simulink model "HANcoder_E407_GTSync_v4"  (R2018b)
settings: Solver=FixedStepDiscrete  StartTime=0.0  StopTime=1  FixedStep=0.01  RelTol=1e-3
PreLoadFcn:
  | librarySetup
  | eval([bdroot,'_startup']) %Calling [modelName]_startup.m
values from neighbouring files (symbols this model uses):
  basic_cycle_duration = TM12 + COMP_duration    (= 495)    [HANcoder_E407_GTSync_v4_startup.m]
  COM_Period = 100    [HANcoder_E407_GTSync_v4_startup.m]
  COM_Phase = COM_Period/2    (= 50)    [HANcoder_E407_GTSync_v4_startup.m]
  comm_delay_estimation = 20    [HANcoder_E407_GTSync_v4_startup.m]
  frequency_IRQ = 20    [HANcoder_E407_GTSync_v4_startup.m]
  HANtuneOverride = Simulink.Parameter    [HANcoder_E407_GTSync_v4_startup.m]
  idle_time_init = basic_cycle_duration*matrix_rows    (= 990)    [HANcoder_E407_GTSync_v4_startup.m]
  LED_ticks_toggle = 10000    [HANcoder_E407_GTSync_v4_startup.m]
  Master_Role = 1    [HANcoder_E407_GTSync_v4_startup.m]
  matrix_rows = 2    [HANcoder_E407_GTSync_v4_startup.m]
  Slave_Role = 2    [HANcoder_E407_GTSync_v4_startup.m]
  Sync_ID = 1    [HANcoder_E407_GTSync_v4_startup.m]
  time_difference_threshold = 500    [HANcoder_E407_GTSync_v4_startup.m]
  TM0 = basic_cycle_start    (= 5)    [HANcoder_E407_GTSync_v4_startup.m]
  TM1 = TM0 + COMM_duration    (= 105)    [HANcoder_E407_GTSync_v4_startup.m]
  TM10 = TM9  + COMP_duration    (= 465)    [HANcoder_E407_GTSync_v4_startup.m]
  TM11 = TM10 + COMP_duration    (= 475)    [HANcoder_E407_GTSync_v4_startup.m]
  TM12 = TM11 + COMP_duration    (= 485)    [HANcoder_E407_GTSync_v4_startup.m]
  TM2 = TM1 + COMP_duration    (= 115)    [HANcoder_E407_GTSync_v4_startup.m]
  TM3 = TM2 + COMP_duration    (= 125)    [HANcoder_E407_GTSync_v4_startup.m]
  TM4 = TM3 + COMM_duration    (= 225)    [HANcoder_E407_GTSync_v4_startup.m]
  TM5 = TM4 + COMP_duration    (= 235)    [HANcoder_E407_GTSync_v4_startup.m]
  TM6 = TM5 + COMM_duration    (= 335)    [HANcoder_E407_GTSync_v4_startup.m]
  TM7 = TM6 + COMP_duration    (= 345)    [HANcoder_E407_GTSync_v4_startup.m]
  TM8 = TM7 + COMM_duration    (= 445)    [HANcoder_E407_GTSync_v4_startup.m]
  TM9 = TM8  + COMP_duration    (= 455)    [HANcoder_E407_GTSync_v4_startup.m]
  Vote1_ID = 12    [HANcoder_E407_GTSync_v4_startup.m]
  Vote2_ID = 22    [HANcoder_E407_GTSync_v4_startup.m]
  Vote3_ID = 32    [HANcoder_E407_GTSync_v4_startup.m]
  wrap_up_threshold = basic_cycle_duration - time_difference_threshold*10    (= -4505)    [HANcoder_E407_GTSync_v4_startup.m]
undefined symbols (not defined in the file or in its folder): A0, A1, CON2
libraries: HANcoder_STM32_Target x22, simulink x3, hdlsllib x2, simulink_extras x1
(part 3 of 5)

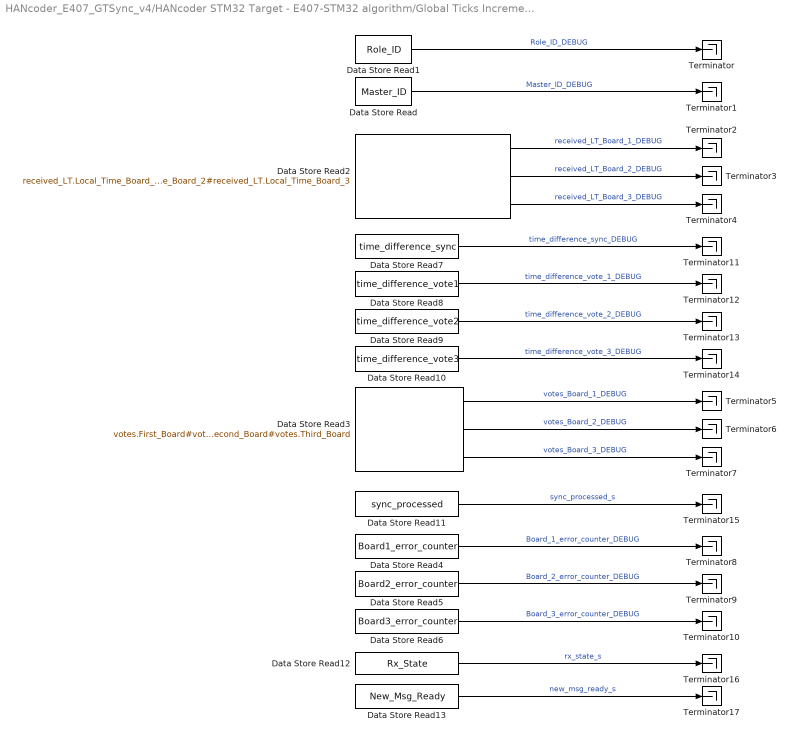
== system HANcoder_E407_GTSync_v4/HANcoder STM32 Target - E407-STM32 algorithm/Global Ticks Increment/CAN Management/Matrix Cycle Manager/Matrix_Cycle_Observation_DEBUG ==
  Data Store Read : DataStoreRead  DataStoreName=Master_ID
  Data Store Read1 : DataStoreRead  DataStoreName=Role_ID
  Data Store Read10 : DataStoreRead  DataStoreName=time_difference_vote3
  Data Store Read11 : DataStoreRead  DataStoreName=sync_processed
  Data Store Read12 : DataStoreRead  DataStoreName=Rx_State
  Data Store Read13 : DataStoreRead  DataStoreName=New_Msg_Ready
  Data Store Read2 : DataStoreRead  DataStoreName=received_LT  DataStoreElements=received_LT.Local_Time_Board_1#received_LT.Local_Time_Board_2#received_LT.Local_Time_Board_3
  Data Store Read3 : DataStoreRead  DataStoreName=votes  DataStoreElements=votes.First_Board#votes.Second_Board#votes.Third_Board
  Data Store Read4 : DataStoreRead  DataStoreName=Board1_error_counter
  Data Store Read5 : DataStoreRead  DataStoreName=Board2_error_counter
  Data Store Read6 : DataStoreRead  DataStoreName=Board3_error_counter
  Data Store Read7 : DataStoreRead  DataStoreName=time_difference_sync
  Data Store Read8 : DataStoreRead  DataStoreName=time_difference_vote1
  Data Store Read9 : DataStoreRead  DataStoreName=time_difference_vote2
  Terminator{,1..17} (18 alike) : Terminator
  wires:
  Data Store Read1/1 -> Terminator/1  "Role_ID_DEBUG"
  Data Store Read/1 -> Terminator1/1  "Master_ID_DEBUG"
  Data Store Read2/1 -> Terminator2/1  "received_LT_Board_1_DEBUG"
  Data Store Read2/2 -> Terminator3/1  "received_LT_Board_2_DEBUG"
  Data Store Read2/3 -> Terminator4/1  "received_LT_Board_3_DEBUG"
  Data Store Read3/1 -> Terminator5/1  "votes_Board_1_DEBUG"
  Data Store Read3/2 -> Terminator6/1  "votes_Board_2_DEBUG"
  Data Store Read3/3 -> Terminator7/1  "votes_Board_3_DEBUG"
  Data Store Read4/1 -> Terminator8/1  "Board_1_error_counter_DEBUG"
  Data Store Read5/1 -> Terminator9/1  "Board_2_error_counter_DEBUG"
  Data Store Read6/1 -> Terminator10/1  "Board_3_error_counter_DEBUG"
  Data Store Read7/1 -> Terminator11/1  "time_difference_sync_DEBUG"
  Data Store Read8/1 -> Terminator12/1  "time_difference_vote_1_DEBUG"
  Data Store Read9/1 -> Terminator13/1  "time_difference_vote_2_DEBUG"
  Data Store Read10/1 -> Terminator14/1  "time_difference_vote_3_DEBUG"
  Data Store Read11/1 -> Terminator15/1  "sync_processed_s"
  Data Store Read12/1 -> Terminator16/1  "rx_state_s"
  Data Store Read13/1 -> Terminator17/1  "new_msg_ready_s"

== system HANcoder_E407_GTSync_v4/HANcoder STM32 Target - E407-STM32 algorithm/Global Ticks Increment/CAN Recieve/RxID_CAN/Sync_ID_CAN ==
  Enable : EnablePort
  CAN receive : Subsystem  Tag=HANcoder_TARGET_STM32_E407  AncestorBlock=HANcoder_STM32_Target/STM32-E407/CAN/CAN/CAN receive  mask(CAN receive){canBus=CAN 2, outputNumber=8, dataType=uint8, byteOrder=off, tsamp=-1}
      mask prompts: canBus "CAN channel"; outputNumber "Output ports"; dataType "Output datatype"; byteOrder "Byte order: Checked = MSB first, unchecked = LSB first."; tsamp "Sample time"
      mask help:
      | Function
      | ==========
      | Receive the newest message from the specified CAN channel.
      |
      | Parameters
      | ==========
      | CAN channel:             The CAN channel to send the message on.
      | Output ports:             The amount of output ports
      | Output datatype:       The datatype of the output ports
      | Byte order:                 Select MSB or LSB first
      | Sample time:              -1 or divisible by base sample time [seconds]
      |
      | Input
      | ==========
      | Port 1:                       CAN ID(uint32) in hexadecimal ie: hex2dec('0a')
      |
      | Output
      | ==========
      | Port 1:                       Checks for new message(int8)
      | Port 2..9                     Message data
      mask init:
      | sfcn_can_receive_mcb(canBus, outputNumber, dataType, byteOrder)
      settings: MoveFcn=drawLogos
      mask Help: web('sfcn_can_receive.html');
      mask TypeOptions canBus: CAN 1 | CAN 2
      mask TypeOptions dataType: int8 | uint8 | int16 | uint16 | int32 | uint32 | boolean
      mask Display:
      | fprintf('Receive on\nCAN %x', canBus);
      | port_label('output', 1, 'new');
      | port_label('input', 1, 'ID');patch([135 141 141],[8 14 2],[1 0 0]);patch([143 143 149],[14 2 8],[0 0 0.35]);
  Constant : Constant  Value=Sync_ID  OutDataTypeStr=uint32
  CAN_new : Outport  OutputWhenDisabled=reset  InitialOutput=0
  Out2 : Outport  Port=2  OutputWhenDisabled=reset  InitialOutput=0
  Out3 : Outport  Port=3  OutputWhenDisabled=reset  InitialOutput=0
  Out4 : Outport  Port=4  OutputWhenDisabled=reset  InitialOutput=0
  Out5 : Outport  Port=5  OutputWhenDisabled=reset  InitialOutput=0
  Out6 : Outport  Port=6  OutputWhenDisabled=reset  InitialOutput=0
  Out7 : Outport  Port=7  OutputWhenDisabled=reset  InitialOutput=0
  Out8 : Outport  Port=8  OutputWhenDisabled=reset  InitialOutput=0
  Out9 : Outport  Port=9  OutputWhenDisabled=reset  InitialOutput=0
  wires:
  CAN receive/1(Out1) -> CAN_new/1
  CAN receive/8(Out8) -> Out8/1
  CAN receive/3(Out3) -> Out3/1
  Constant/1 -> CAN receive/1(In1)
  CAN receive/2(Out2) -> Out2/1
  CAN receive/6(Out6) -> Out6/1
  CAN receive/7(Out7) -> Out7/1
  CAN receive/4(Out4) -> Out4/1
  CAN receive/5(Out5) -> Out5/1
  CAN receive/9(Out9) -> Out9/1

== system HANcoder_E407_GTSync_v4/HANcoder STM32 Target - E407-STM32 algorithm/Global Ticks Increment/CAN Recieve/RxID_CAN/Vote1_ID_CAN ==
  Enable : EnablePort
  CAN receive : Subsystem  Tag=HANcoder_TARGET_STM32_E407  AncestorBlock=HANcoder_STM32_Target/STM32-E407/CAN/CAN/CAN receive  mask(CAN receive){canBus=CAN 2, outputNumber=8, dataType=uint8, byteOrder=off, tsamp=-1}
      mask prompts: canBus "CAN channel"; outputNumber "Output ports"; dataType "Output datatype"; byteOrder "Byte order: Checked = MSB first, unchecked = LSB first."; tsamp "Sample time"
      mask help:
      | Function
      | ==========
      | Receive the newest message from the specified CAN channel.
      |
      | Parameters
      | ==========
      | CAN channel:             The CAN channel to send the message on.
      | Output ports:             The amount of output ports
      | Output datatype:       The datatype of the output ports
      | Byte order:                 Select MSB or LSB first
      | Sample time:              -1 or divisible by base sample time [seconds]
      |
      | Input
      | ==========
      | Port 1:                       CAN ID(uint32) in hexadecimal ie: hex2dec('0a')
      |
      | Output
      | ==========
      | Port 1:                       Checks for new message(int8)
      | Port 2..9                     Message data
      mask init:
      | sfcn_can_receive_mcb(canBus, outputNumber, dataType, byteOrder)
      settings: MoveFcn=drawLogos
      mask Help: web('sfcn_can_receive.html');
      mask TypeOptions canBus: CAN 1 | CAN 2
      mask TypeOptions dataType: int8 | uint8 | int16 | uint16 | int32 | uint32 | boolean
      mask Display:
      | fprintf('Receive on\nCAN %x', canBus);
      | port_label('output', 1, 'new');
      | port_label('input', 1, 'ID');patch([135 141 141],[8 14 2],[1 0 0]);patch([143 143 149],[14 2 8],[0 0 0.35]);
  Constant : Constant  Value=Vote1_ID  OutDataTypeStr=uint32
  CAN_new : Outport  OutputWhenDisabled=reset  InitialOutput=0
  Out2 : Outport  Port=2  OutputWhenDisabled=reset  InitialOutput=0
  Out3 : Outport  Port=3  OutputWhenDisabled=reset  InitialOutput=0
  Out4 : Outport  Port=4  OutputWhenDisabled=reset  InitialOutput=0
  Out5 : Outport  Port=5  OutputWhenDisabled=reset  InitialOutput=0
  Out6 : Outport  Port=6  OutputWhenDisabled=reset  InitialOutput=0
  Out7 : Outport  Port=7  OutputWhenDisabled=reset  InitialOutput=0
  Out8 : Outport  Port=8  OutputWhenDisabled=reset  InitialOutput=0
  Out9 : Outport  Port=9  OutputWhenDisabled=reset  InitialOutput=0
  wires:
  CAN receive/9(Out9) -> Out9/1
  CAN receive/5(Out5) -> Out5/1
  CAN receive/4(Out4) -> Out4/1
  CAN receive/7(Out7) -> Out7/1
  CAN receive/6(Out6) -> Out6/1
  CAN receive/2(Out2) -> Out2/1
  Constant/1 -> CAN receive/1(In1)
  CAN receive/3(Out3) -> Out3/1
  CAN receive/8(Out8) -> Out8/1
  CAN receive/1(Out1) -> CAN_new/1

== system HANcoder_E407_GTSync_v4/HANcoder STM32 Target - E407-STM32 algorithm/Global Ticks Increment/CAN Recieve/RxID_CAN/Vote2_ID_CAN ==
  Enable : EnablePort
  CAN receive : Subsystem  Tag=HANcoder_TARGET_STM32_E407  AncestorBlock=HANcoder_STM32_Target/STM32-E407/CAN/CAN/CAN receive  mask(CAN receive){canBus=CAN 2, outputNumber=8, dataType=uint8, byteOrder=off, tsamp=-1}
      mask prompts: canBus "CAN channel"; outputNumber "Output ports"; dataType "Output datatype"; byteOrder "Byte order: Checked = MSB first, unchecked = LSB first."; tsamp "Sample time"
      mask help:
      | Function
      | ==========
      | Receive the newest message from the specified CAN channel.
      |
      | Parameters
      | ==========
      | CAN channel:             The CAN channel to send the message on.
      | Output ports:             The amount of output ports
      | Output datatype:       The datatype of the output ports
      | Byte order:                 Select MSB or LSB first
      | Sample time:              -1 or divisible by base sample time [seconds]
      |
      | Input
      | ==========
      | Port 1:                       CAN ID(uint32) in hexadecimal ie: hex2dec('0a')
      |
      | Output
      | ==========
      | Port 1:                       Checks for new message(int8)
      | Port 2..9                     Message data
      mask init:
      | sfcn_can_receive_mcb(canBus, outputNumber, dataType, byteOrder)
      settings: MoveFcn=drawLogos
      mask Help: web('sfcn_can_receive.html');
      mask TypeOptions canBus: CAN 1 | CAN 2
      mask TypeOptions dataType: int8 | uint8 | int16 | uint16 | int32 | uint32 | boolean
      mask Display:
      | fprintf('Receive on\nCAN %x', canBus);
      | port_label('output', 1, 'new');
      | port_label('input', 1, 'ID');patch([135 141 141],[8 14 2],[1 0 0]);patch([143 143 149],[14 2 8],[0 0 0.35]);
  Constant : Constant  Value=Vote2_ID  OutDataTypeStr=uint32
  CAN_new : Outport  OutputWhenDisabled=reset  InitialOutput=0
  Out2 : Outport  Port=2  OutputWhenDisabled=reset  InitialOutput=0
  Out3 : Outport  Port=3  OutputWhenDisabled=reset  InitialOutput=0
  Out4 : Outport  Port=4  OutputWhenDisabled=reset  InitialOutput=0
  Out5 : Outport  Port=5  OutputWhenDisabled=reset  InitialOutput=0
  Out6 : Outport  Port=6  OutputWhenDisabled=reset  InitialOutput=0
  Out7 : Outport  Port=7  OutputWhenDisabled=reset  InitialOutput=0
  Out8 : Outport  Port=8  OutputWhenDisabled=reset  InitialOutput=0
  Out9 : Outport  Port=9  OutputWhenDisabled=reset  InitialOutput=0
  wires:
  CAN receive/1(Out1) -> CAN_new/1
  CAN receive/8(Out8) -> Out8/1
  CAN receive/3(Out3) -> Out3/1
  Constant/1 -> CAN receive/1(In1)
  CAN receive/2(Out2) -> Out2/1
  CAN receive/6(Out6) -> Out6/1
  CAN receive/7(Out7) -> Out7/1
  CAN receive/4(Out4) -> Out4/1
  CAN receive/5(Out5) -> Out5/1
  CAN receive/9(Out9) -> Out9/1

== system HANcoder_E407_GTSync_v4/HANcoder STM32 Target - E407-STM32 algorithm/Global Ticks Increment/CAN Recieve/RxID_CAN/Vote3_ID_CAN ==
  Enable : EnablePort
  CAN receive : Subsystem  Tag=HANcoder_TARGET_STM32_E407  AncestorBlock=HANcoder_STM32_Target/STM32-E407/CAN/CAN/CAN receive  mask(CAN receive){canBus=CAN 2, outputNumber=8, dataType=uint8, byteOrder=off, tsamp=-1}
      mask prompts: canBus "CAN channel"; outputNumber "Output ports"; dataType "Output datatype"; byteOrder "Byte order: Checked = MSB first, unchecked = LSB first."; tsamp "Sample time"
      mask help:
      | Function
      | ==========
      | Receive the newest message from the specified CAN channel.
      |
      | Parameters
      | ==========
      | CAN channel:             The CAN channel to send the message on.
      | Output ports:             The amount of output ports
      | Output datatype:       The datatype of the output ports
      | Byte order:                 Select MSB or LSB first
      | Sample time:              -1 or divisible by base sample time [seconds]
      |
      | Input
      | ==========
      | Port 1:                       CAN ID(uint32) in hexadecimal ie: hex2dec('0a')
      |
      | Output
      | ==========
      | Port 1:                       Checks for new message(int8)
      | Port 2..9                     Message data
      mask init:
      | sfcn_can_receive_mcb(canBus, outputNumber, dataType, byteOrder)
      settings: MoveFcn=drawLogos
      mask Help: web('sfcn_can_receive.html');
      mask TypeOptions canBus: CAN 1 | CAN 2
      mask TypeOptions dataType: int8 | uint8 | int16 | uint16 | int32 | uint32 | boolean
      mask Display:
      | fprintf('Receive on\nCAN %x', canBus);
      | port_label('output', 1, 'new');
      | port_label('input', 1, 'ID');patch([135 141 141],[8 14 2],[1 0 0]);patch([143 143 149],[14 2 8],[0 0 0.35]);
  Constant : Constant  Value=Vote3_ID  OutDataTypeStr=uint32
  CAN_new : Outport  OutputWhenDisabled=reset  InitialOutput=0
  Out2 : Outport  Port=2  OutputWhenDisabled=reset  InitialOutput=0
  Out3 : Outport  Port=3  OutputWhenDisabled=reset  InitialOutput=0
  Out4 : Outport  Port=4  OutputWhenDisabled=reset  InitialOutput=0
  Out5 : Outport  Port=5  OutputWhenDisabled=reset  InitialOutput=0
  Out6 : Outport  Port=6  OutputWhenDisabled=reset  InitialOutput=0
  Out7 : Outport  Port=7  OutputWhenDisabled=reset  InitialOutput=0
  Out8 : Outport  Port=8  OutputWhenDisabled=reset  InitialOutput=0
  Out9 : Outport  Port=9  OutputWhenDisabled=reset  InitialOutput=0
  wires:
  CAN receive/9(Out9) -> Out9/1
  CAN receive/5(Out5) -> Out5/1
  CAN receive/4(Out4) -> Out4/1
  CAN receive/7(Out7) -> Out7/1
  CAN receive/6(Out6) -> Out6/1
  CAN receive/2(Out2) -> Out2/1
  Constant/1 -> CAN receive/1(In1)
  CAN receive/3(Out3) -> Out3/1
  CAN receive/8(Out8) -> Out8/1
  CAN receive/1(Out1) -> CAN_new/1

== system HANcoder_E407_GTSync_v4/HANcoder STM32 Target - E407-STM32 algorithm/Global Ticks Increment/CAN Recieve/Update message buffers/UINT8 to UINT16 ==
  In1 : Inport
  In2 : Inport  Port=2
  Bit Shift : hdlsllib/Logic and Bit Operations/Bit Shift  mode=Shift Left Logical  N=8
      settings: SourceProductName=HDL Coder  SourceProductBaseCode=HD
  Cast1 : DataTypeConversion  OutDataTypeStr=uint16
  Cast4 : DataTypeConversion  OutDataTypeStr=uint16
  Sum1 : Sum
  Out1 : Outport
  wires:
  In1/1 -> Cast4/1
  Bit Shift/1 -> Sum1/2
  Cast1/1 -> Bit Shift/1
  In2/1 -> Cast1/1
  Sum1/1 -> Out1/1
  Cast4/1 -> Sum1/1

== system HANcoder_E407_GTSync_v4/HANcoder STM32 Target - E407-STM32 algorithm/Global Ticks Increment/CAN Management/Initialization/Delay/Initializaton_Observation_DEBUG ==
  Data Store Read : DataStoreRead  DataStoreName=Initialization_flag
  Data Store Read1 : DataStoreRead  DataStoreName=Delay_Counter
  Data Store Read2 : DataStoreRead  DataStoreName=New_Msg_Ready
  Data Store Read3 : DataStoreRead  DataStoreName=Initialization_Timeout
  Data Store Read5 : DataStoreRead  DataStoreName=basic_cycle_count
  Terminator{,1..3,5} (5 alike) : Terminator
  wires:
  Data Store Read3/1 -> Terminator3/1  "initialization_timeout_DEBUG"
  Data Store Read1/1 -> Terminator1/1  "delay_counter_DEBUG"
  Data Store Read/1 -> Terminator/1  "initialization_flag_DEBUG"
  Data Store Read5/1 -> Terminator5/1  "basic_cycle_DEBUG"
  Data Store Read2/1 -> Terminator2/1  "New_Msg_Rx_DEBUG"

== system HANcoder_E407_GTSync_v4/HANcoder STM32 Target - E407-STM32 algorithm/Global Ticks Increment/CAN Management/Initialization/RoleID and Global Time init/Global Time Initialization Master ==
  note: Global Time Initialization
  Enable : EnablePort
  Board nr1 : Constant
  Data Store Write3 : DataStoreWrite  DataStoreName=Master_ID
  wires:
  Board nr1/1 -> Data Store Write3/1

== system HANcoder_E407_GTSync_v4/HANcoder STM32 Target - E407-STM32 algorithm/Global Ticks Increment/CAN Management/Initialization/RoleID and Global Time init/Global Time Initialization Slave ==
  note: Global Time Initialization
  Enable : EnablePort
  Data Store Read1 : DataStoreRead  DataStoreName=Local_Ticks_Rx
  Data Store Read2 : DataStoreRead  DataStoreName=Basic_Cycle_Rx
  Data Store Read3 : DataStoreRead  DataStoreName=Msg_Header_Rx
  Data Store Write1 : DataStoreWrite  DataStoreName=Local_Ticks
  Data Store Write2 : DataStoreWrite  DataStoreName=basic_cycle_count
  Data Store Write3 : DataStoreWrite  DataStoreName=Master_ID
  wires:
  Data Store Read1/1 -> Data Store Write1/1
  Data Store Read3/1 -> Data Store Write3/1
  Data Store Read2/1 -> Data Store Write2/1

== system HANcoder_E407_GTSync_v4/HANcoder STM32 Target - E407-STM32 algorithm/Global Ticks Increment/CAN Management/Matrix Cycle Manager/COM Task - Sync BC0/Sync Msg ==
  note: Reset Rx buffers
  note: Wait until new message
      | arrives
  note: Message Data (2)
      |    Basic cycle for Sync
  note: Basic Cycle 0
      | Time Window 0
      | Message Sent: < Only if RoleID == 1 (Master) >
      | 	TxMessage ID: Sync
      | 	Message Header: BoardID
      | 	Message buffert : Local Time
      | Message Receive: < Only if RoleID ~= 1 (Slave)>
      | 	RxMessage ID: Sync
  note: Message Data
      |    Every message sends
      |    Local_Time as Data
  note: Transmission ID
      |    Sync Msg: 1
      |    Vote Node 1: 12
      |    Vote Node 2: 22
      |    Vote Node 3: 32
  note: Message Information
      |    Sync: BoardID
      |    Vote: Vote information
  note: Reception ID
      |    Sync Msg: 1
      |    Vote Node 1: 12
      |    Vote Node 2: 22
      |    Vote Node 3: 32
  note: Reset RX Buffer Flag
  Enable : EnablePort
  Cast : DataTypeConversion  OutDataTypeStr=uint32
  Cast1 : DataTypeConversion  OutDataTypeStr=uint16
  Cast2 : DataTypeConversion  OutDataTypeStr=uint8
  Cast3 : DataTypeConversion  OutDataTypeStr=uint32
  Cast4 : DataTypeConversion  OutDataTypeStr=uint8
  Cast5 : DataTypeConversion  OutDataTypeStr=boolean
  Cast6 : DataTypeConversion  OutDataTypeStr=uint8
  Constant : Constant  Value=Sync_ID
  Constant1 : Constant  Value=comm_delay_estimation
  Constant18 : Constant  Value=COM_Phase
  Constant2 : Constant  Value=Sync_ID
  Data Store Read : DataStoreRead  DataStoreName=Local_Ticks
  Data Store Read2 : DataStoreRead  DataStoreName=Board_ID
  Data Store Read3 : DataStoreRead  DataStoreName=basic_cycle_count
  Data Store Write : DataStoreWrite  DataStoreName=Msg_Header_Rx
  Data Store Write1 : DataStoreWrite  DataStoreName=basic_cycle_buffer
  Data Store Write2 : DataStoreWrite  DataStoreName=New_Msg_Ready
  Data Store Write3 : DataStoreWrite  DataStoreName=Local_Ticks_Rx
  Data Store Write4 : DataStoreWrite  DataStoreName=Basic_Cycle_Rx
  Data Store Write5 : DataStoreWrite  DataStoreName=message_header_buffer
  Data Store Write6 : DataStoreWrite  DataStoreName=RxID_buffer
  Data Store Write7 : DataStoreWrite  DataStoreName=Rx_State
  Data Store Write8 : DataStoreWrite  DataStoreName=TxID_buffer
  Data Store Write9 : DataStoreWrite  DataStoreName=local_ticks_buffer
  Minus1 : Sum  Inputs=+++
  RESET : Constant  Value=0
  RESET_CAN_new_buffer : Constant  Value=0
  RESET_Rx_BC : Constant  Value=0  OutDataTypeStr=uint8
  RESET_Rx_Hdr : Constant  Value=0
  RESET_Rx_LT : Constant  Value=0  OutDataTypeStr=uint16
  wires:
  Constant18/1 -> Minus1/2
  Minus1/1 -> Cast1/1
  Cast1/1 -> Data Store Write9/1
  Cast/1 -> Data Store Write8/1
  Data Store Read/1 -> Minus1/1
  Constant/1 -> Cast/1
  Cast3/1 -> Data Store Write6/1
  Constant2/1 -> Cast3/1
  Cast2/1 -> Data Store Write5/1
  Cast4/1 -> Data Store Write1/1
  Data Store Read3/1 -> Cast4/1
  Data Store Read2/1 -> Cast2/1
  RESET/1 -> Cast5/1
  Cast5/1 -> Data Store Write2/1
  RESET_Rx_Hdr/1 -> Data Store Write/1
  RESET_Rx_LT/1 -> Data Store Write3/1
  RESET_Rx_BC/1 -> Data Store Write4/1
  RESET_CAN_new_buffer/1 -> Cast6/1
  Cast6/1 -> Data Store Write7/1
  Constant1/1 -> Minus1/3

== system HANcoder_E407_GTSync_v4/HANcoder STM32 Target - E407-STM32 algorithm/Global Ticks Increment/CAN Management/Matrix Cycle Manager/COM Task - Sync BC1/Sync Msg ==
  note: Reset Rx buffers
  note: Wait until new message
      | arrives
  note: Message Data (2)
      |    Basic cycle for Sync
  note: Basic Cycle 0
      | Time Window 0
      | Message Sent: < Only if RoleID == 1 (Master) >
      | 	TxMessage ID: Sync
      | 	Message Header: BoardID
      | 	Message buffert : Local Time
      | Message Receive: < Only if RoleID ~= 1 (Slave)>
      | 	RxMessage ID: Sync
  note: Message Data
      |    Every message sends
      |    Local_Time as Data
  note: Transmission ID
      |    Sync Msg: 1
      |    Vote Node 1: 12
      |    Vote Node 2: 22
      |    Vote Node 3: 32
  note: Message Information
      |    Sync: BoardID
      |    Vote: Vote information
  note: Reception ID
      |    Sync Msg: 1
      |    Vote Node 1: 12
      |    Vote Node 2: 22
      |    Vote Node 3: 32
  note: Reset RX Buffer Flag
  Enable : EnablePort
  Cast : DataTypeConversion  OutDataTypeStr=uint32
  Cast1 : DataTypeConversion  OutDataTypeStr=uint16
  Cast2 : DataTypeConversion  OutDataTypeStr=uint8
  Cast3 : DataTypeConversion  OutDataTypeStr=uint32
  Cast4 : DataTypeConversion  OutDataTypeStr=uint8
  Cast5 : DataTypeConversion  OutDataTypeStr=boolean
  Cast6 : DataTypeConversion  OutDataTypeStr=uint8
  Constant : Constant  Value=Sync_ID
  Constant18 : Constant  Value=COM_Phase
  Constant2 : Constant  Value=Sync_ID
  Data Store Read : DataStoreRead  DataStoreName=Local_Ticks
  Data Store Read2 : DataStoreRead  DataStoreName=Board_ID
  Data Store Read3 : DataStoreRead  DataStoreName=basic_cycle_count
  Data Store Write : DataStoreWrite  DataStoreName=Msg_Header_Rx
  Data Store Write1 : DataStoreWrite  DataStoreName=basic_cycle_buffer
  Data Store Write2 : DataStoreWrite  DataStoreName=New_Msg_Ready
  Data Store Write3 : DataStoreWrite  DataStoreName=Local_Ticks_Rx
  Data Store Write4 : DataStoreWrite  DataStoreName=Basic_Cycle_Rx
  Data Store Write5 : DataStoreWrite  DataStoreName=message_header_buffer
  Data Store Write6 : DataStoreWrite  DataStoreName=RxID_buffer
  Data Store Write7 : DataStoreWrite  DataStoreName=Rx_State
  Data Store Write8 : DataStoreWrite  DataStoreName=TxID_buffer
  Data Store Write9 : DataStoreWrite  DataStoreName=local_ticks_buffer
  Minus1 : Sum
  RESET : Constant  Value=0
  RESET_CAN_new_buffer : Constant  Value=0
  RESET_Rx_BC : Constant  Value=0  OutDataTypeStr=uint8
  RESET_Rx_Hdr : Constant  Value=0
  RESET_Rx_LT : Constant  Value=0  OutDataTypeStr=uint16
  wires:
  Constant18/1 -> Minus1/2
  Minus1/1 -> Cast1/1
  Cast1/1 -> Data Store Write9/1
  Cast/1 -> Data Store Write8/1
  Constant/1 -> Cast/1
  Cast3/1 -> Data Store Write6/1
  Constant2/1 -> Cast3/1
  Cast2/1 -> Data Store Write5/1
  Cast4/1 -> Data Store Write1/1
  Data Store Read3/1 -> Cast4/1
  Data Store Read2/1 -> Cast2/1
  RESET/1 -> Cast5/1
  Cast5/1 -> Data Store Write2/1
  RESET_Rx_Hdr/1 -> Data Store Write/1
  RESET_Rx_LT/1 -> Data Store Write3/1
  RESET_Rx_BC/1 -> Data Store Write4/1
  Cast6/1 -> Data Store Write7/1
  RESET_CAN_new_buffer/1 -> Cast6/1
  Data Store Read/1 -> Minus1/1

== system HANcoder_E407_GTSync_v4/HANcoder STM32 Target - E407-STM32 algorithm/Global Ticks Increment/CAN Management/Matrix Cycle Manager/COM Task - Vote1/Vote1 Msg ==
  note: Reception ID
      |    Sync Msg: 1
      |    Vote Node 1: 12
      |    Vote Node 2: 22
      |    Vote Node 3: 32
  note: Message Information
      |    Sync: BoardID
      |    Vote: Vote information
  note: Transmission ID
      |    Sync Msg: 1
      |    Vote Node 1: 12
      |    Vote Node 2: 22
      |    Vote Node 3: 32
  note: Message Data
      |    Every message sends
      |    Local_Time as Data
  note: Basic Cycle 0
      | Time Window 1
      | Message Sent: < Only if BoardID == 1 >
      | 	TxMessage ID: Vote1
      | 	Message Header: Vote
      | 	Message buffert : Local Time
      | Message Receive: < Only if BoardID ~= 1 >
      | 	RxMessage ID: Vote1
  note: Message Data (2)
      |    Basic cycle for Sync
  note: Wait until new message
      | arrives
  note: Reset Rx buffers
  note: Reset RX Buffer Flag
  Enable : EnablePort
  Cast : DataTypeConversion  OutDataTypeStr=uint32
  Cast1 : DataTypeConversion  OutDataTypeStr=uint16
  Cast3 : DataTypeConversion  OutDataTypeStr=uint32
  Cast4 : DataTypeConversion  OutDataTypeStr=uint8
  Cast5 : DataTypeConversion  OutDataTypeStr=boolean
  Cast6 : DataTypeConversion  OutDataTypeStr=uint8
  Constant : Constant  Value=Vote1_ID
  Constant18 : Constant  Value=COM_Phase
  Constant2 : Constant  Value=Vote1_ID
  Data Store Read : DataStoreRead  DataStoreName=Local_Ticks
  Data Store Read2 : DataStoreRead  DataStoreName=Vote
  Data Store Read3 : DataStoreRead  DataStoreName=basic_cycle_count
  Data Store Write : DataStoreWrite  DataStoreName=Msg_Header_Rx
  Data Store Write1 : DataStoreWrite  DataStoreName=basic_cycle_buffer
  Data Store Write2 : DataStoreWrite  DataStoreName=New_Msg_Ready
  Data Store Write3 : DataStoreWrite  DataStoreName=Local_Ticks_Rx
  Data Store Write4 : DataStoreWrite  DataStoreName=Basic_Cycle_Rx
  Data Store Write5 : DataStoreWrite  DataStoreName=message_header_buffer
  Data Store Write6 : DataStoreWrite  DataStoreName=RxID_buffer
  Data Store Write7 : DataStoreWrite  DataStoreName=Rx_State
  Data Store Write8 : DataStoreWrite  DataStoreName=TxID_buffer
  Data Store Write9 : DataStoreWrite  DataStoreName=local_ticks_buffer
  Minus1 : Sum
  RESET : Constant  Value=0
  RESET_CAN_new_buffer : Constant  Value=0
  RESET_Rx_BC : Constant  Value=0  OutDataTypeStr=uint8
  RESET_Rx_Hdr : Constant  Value=0
  RESET_Rx_LT : Constant  Value=0  OutDataTypeStr=uint16
  wires:
  Constant2/1 -> Cast3/1
  Cast3/1 -> Data Store Write6/1
  Data Store Read2/1 -> Data Store Write5/1
  Constant/1 -> Cast/1
  Data Store Read/1 -> Minus1/1
  Cast/1 -> Data Store Write8/1
  Cast1/1 -> Data Store Write9/1
  Minus1/1 -> Cast1/1
  Constant18/1 -> Minus1/2
  Data Store Read3/1 -> Cast4/1
  Cast4/1 -> Data Store Write1/1
  RESET/1 -> Cast5/1
  Cast5/1 -> Data Store Write2/1
  RESET_Rx_LT/1 -> Data Store Write3/1
  RESET_Rx_BC/1 -> Data Store Write4/1
  RESET_Rx_Hdr/1 -> Data Store Write/1
  Cast6/1 -> Data Store Write7/1
  RESET_CAN_new_buffer/1 -> Cast6/1

== system HANcoder_E407_GTSync_v4/HANcoder STM32 Target - E407-STM32 algorithm/Global Ticks Increment/CAN Management/Matrix Cycle Manager/COM Task - Vote2/Vote2 Msg ==
  note: Basic Cycle 0
      | Time Window 2
      | Message Sent: < Only if BoardID == 2 >
      | 	TxMessage ID: Vote2
      | 	Message Header: Vote
      | 	Message buffert : Local Time
      | Message Receive: < Only if BoardID ~= 2 >
      | 	RxMessage ID: Vote2
  note: Message Data
      |    Every message sends
      |    Local_Time as Data
  note: Transmission ID
      |    Sync Msg: 1
      |    Vote Node 1: 12
      |    Vote Node 2: 22
      |    Vote Node 3: 32
  note: Message Information
      |    Sync: BoardID
      |    Vote: Vote information
  note: Reception ID
      |    Sync Msg: 1
      |    Vote Node 1: 12
      |    Vote Node 2: 22
      |    Vote Node 3: 32
  note: Message Data (2)
      |    Basic cycle for Sync
  note: Wait until new message
      | arrives
  note: Reset Rx buffers
  note: Reset RX Buffer Flag
  Enable : EnablePort
  Cast : DataTypeConversion  OutDataTypeStr=uint32
  Cast1 : DataTypeConversion  OutDataTypeStr=uint16
  Cast3 : DataTypeConversion  OutDataTypeStr=uint32
  Cast4 : DataTypeConversion  OutDataTypeStr=uint8
  Cast5 : DataTypeConversion  OutDataTypeStr=boolean
  Cast6 : DataTypeConversion  OutDataTypeStr=uint8
  Constant : Constant  Value=Vote2_ID
  Constant18 : Constant  Value=COM_Phase
  Constant2 : Constant  Value=Vote2_ID
  Data Store Read : DataStoreRead  DataStoreName=Local_Ticks
  Data Store Read2 : DataStoreRead  DataStoreName=Vote
  Data Store Read3 : DataStoreRead  DataStoreName=basic_cycle_count
  Data Store Write : DataStoreWrite  DataStoreName=Msg_Header_Rx
  Data Store Write1 : DataStoreWrite  DataStoreName=basic_cycle_buffer
  Data Store Write2 : DataStoreWrite  DataStoreName=New_Msg_Ready
  Data Store Write3 : DataStoreWrite  DataStoreName=Local_Ticks_Rx
  Data Store Write4 : DataStoreWrite  DataStoreName=Basic_Cycle_Rx
  Data Store Write5 : DataStoreWrite  DataStoreName=message_header_buffer
  Data Store Write6 : DataStoreWrite  DataStoreName=RxID_buffer
  Data Store Write7 : DataStoreWrite  DataStoreName=Rx_State
  Data Store Write8 : DataStoreWrite  DataStoreName=TxID_buffer
  Data Store Write9 : DataStoreWrite  DataStoreName=local_ticks_buffer
  Minus1 : Sum
  RESET : Constant  Value=0
  RESET_CAN_new_buffer : Constant  Value=0
  RESET_Rx_BC : Constant  Value=0  OutDataTypeStr=uint8
  RESET_Rx_Hdr : Constant  Value=0
  RESET_Rx_LT : Constant  Value=0  OutDataTypeStr=uint16
  wires:
  Constant18/1 -> Minus1/2
  Minus1/1 -> Cast1/1
  Cast1/1 -> Data Store Write9/1
  Cast/1 -> Data Store Write8/1
  Data Store Read/1 -> Minus1/1
  Constant/1 -> Cast/1
  Data Store Read2/1 -> Data Store Write5/1
  Cast3/1 -> Data Store Write6/1
  Constant2/1 -> Cast3/1
  Data Store Read3/1 -> Cast4/1
  Cast4/1 -> Data Store Write1/1
  RESET/1 -> Cast5/1
  Cast5/1 -> Data Store Write2/1
  RESET_Rx_LT/1 -> Data Store Write3/1
  RESET_Rx_BC/1 -> Data Store Write4/1
  RESET_Rx_Hdr/1 -> Data Store Write/1
  Cast6/1 -> Data Store Write7/1
  RESET_CAN_new_buffer/1 -> Cast6/1

== system HANcoder_E407_GTSync_v4/HANcoder STM32 Target - E407-STM32 algorithm/Global Ticks Increment/CAN Management/Matrix Cycle Manager/COM Task - Vote3/Vote3 Msg ==
  note: Reception ID
      |    Sync Msg: 1
      |    Vote Node 1: 12
      |    Vote Node 2: 22
      |    Vote Node 3: 32
  note: Message Information
      |    Sync: BoardID
      |    Vote: Vote information
  note: Transmission ID
      |    Sync Msg: 1
      |    Vote Node 1: 12
      |    Vote Node 2: 22
      |    Vote Node 3: 32
  note: Message Data
      |    Every message sends
      |    Local_Time as Data
  note: Basic Cycle 0
      | Time Window 3
      | Message Sent: < Only if BoardID == 3 >
      | 	TxMessage ID: Vote3
      | 	Message Header: Vote
      | 	Message buffert : Local Time
      | Message Receive: < Only if BoardID ~= 3 >
      | 	RxMessage ID: Vote3
  note: Message Data (2)
      |    Basic cycle for Sync
  note: Wait until new message
      | arrives
  note: Reset Rx buffers
  note: Reset RX Buffer Flag
  Enable : EnablePort
  Cast : DataTypeConversion  OutDataTypeStr=uint32
  Cast1 : DataTypeConversion  OutDataTypeStr=uint16
  Cast3 : DataTypeConversion  OutDataTypeStr=uint32
  Cast4 : DataTypeConversion  OutDataTypeStr=uint8
  Cast5 : DataTypeConversion  OutDataTypeStr=boolean
  Cast6 : DataTypeConversion  OutDataTypeStr=uint8
  Constant : Constant  Value=Vote3_ID
  Constant18 : Constant  Value=COM_Phase
  Constant2 : Constant  Value=Vote3_ID
  Data Store Read : DataStoreRead  DataStoreName=Local_Ticks
  Data Store Read2 : DataStoreRead  DataStoreName=Vote
  Data Store Read3 : DataStoreRead  DataStoreName=basic_cycle_count
  Data Store Write : DataStoreWrite  DataStoreName=Msg_Header_Rx
  Data Store Write1 : DataStoreWrite  DataStoreName=basic_cycle_buffer
  Data Store Write2 : DataStoreWrite  DataStoreName=New_Msg_Ready
  Data Store Write3 : DataStoreWrite  DataStoreName=Local_Ticks_Rx
  Data Store Write4 : DataStoreWrite  DataStoreName=Basic_Cycle_Rx
  Data Store Write5 : DataStoreWrite  DataStoreName=message_header_buffer
  Data Store Write6 : DataStoreWrite  DataStoreName=RxID_buffer
  Data Store Write7 : DataStoreWrite  DataStoreName=Rx_State
  Data Store Write8 : DataStoreWrite  DataStoreName=TxID_buffer
  Data Store Write9 : DataStoreWrite  DataStoreName=local_ticks_buffer
  Minus1 : Sum
  RESET : Constant  Value=0
  RESET_CAN_new_buffer : Constant  Value=0
  RESET_Rx_BC : Constant  Value=0  OutDataTypeStr=uint8
  RESET_Rx_Hdr : Constant  Value=0
  RESET_Rx_LT : Constant  Value=0  OutDataTypeStr=uint16
  wires:
  Constant2/1 -> Cast3/1
  Cast3/1 -> Data Store Write6/1
  Data Store Read2/1 -> Data Store Write5/1
  Constant/1 -> Cast/1
  Data Store Read/1 -> Minus1/1
  Cast/1 -> Data Store Write8/1
  Cast1/1 -> Data Store Write9/1
  Minus1/1 -> Cast1/1
  Constant18/1 -> Minus1/2
  Data Store Read3/1 -> Cast4/1
  Cast4/1 -> Data Store Write1/1
  RESET/1 -> Cast5/1
  Cast5/1 -> Data Store Write2/1
  RESET_Rx_LT/1 -> Data Store Write3/1
  RESET_Rx_BC/1 -> Data Store Write4/1
  RESET_Rx_Hdr/1 -> Data Store Write/1
  Cast6/1 -> Data Store Write7/1
  RESET_CAN_new_buffer/1 -> Cast6/1

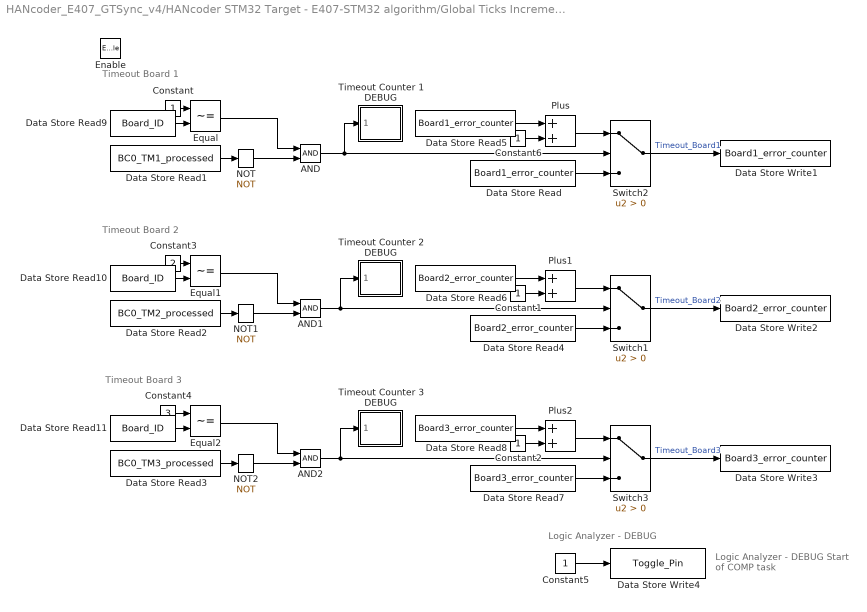
== system HANcoder_E407_GTSync_v4/HANcoder STM32 Target - E407-STM32 algorithm/Global Ticks Increment/CAN Management/Matrix Cycle Manager/COMP Task - Check Timeouts/Timeout and Board error counter ==
  note: Timeout Board 2
  note: Timeout Board 3
  note: Timeout Board 1
  note: Logic Analyzer - DEBUG
      | Start of COMP task
  note: Logic Analyzer - DEBUG
  Enable : EnablePort  PropagateVarSize=During execution
  AND : Logic  IconShape=distinctive  AllPortsSameDT=off  OutDataTypeStr=boolean
  AND1 : Logic  IconShape=distinctive  AllPortsSameDT=off  OutDataTypeStr=boolean
  AND2 : Logic  IconShape=distinctive  AllPortsSameDT=off  OutDataTypeStr=boolean
  Constant{,1..2,6} (4 alike) : Constant
  Constant3 : Constant  Value=2
  Constant4 : Constant  Value=3
  Constant5 : Constant  OutDataTypeStr=boolean
  Data Store Read : DataStoreRead  DataStoreName=Board1_error_counter
  Data Store Read1 : DataStoreRead  DataStoreName=BC0_TM1_processed
  Data Store Read10 : DataStoreRead  DataStoreName=Board_ID
  Data Store Read11 : DataStoreRead  DataStoreName=Board_ID
  Data Store Read2 : DataStoreRead  DataStoreName=BC0_TM2_processed
  Data Store Read3 : DataStoreRead  DataStoreName=BC0_TM3_processed
  Data Store Read4 : DataStoreRead  DataStoreName=Board2_error_counter
  Data Store Read5 : DataStoreRead  DataStoreName=Board1_error_counter
  Data Store Read6 : DataStoreRead  DataStoreName=Board2_error_counter
  Data Store Read7 : DataStoreRead  DataStoreName=Board3_error_counter
  Data Store Read8 : DataStoreRead  DataStoreName=Board3_error_counter
  Data Store Read9 : DataStoreRead  DataStoreName=Board_ID
  Data Store Write1 : DataStoreWrite  DataStoreName=Board1_error_counter
  Data Store Write2 : DataStoreWrite  DataStoreName=Board2_error_counter
  Data Store Write3 : DataStoreWrite  DataStoreName=Board3_error_counter
  Data Store Write4 : DataStoreWrite  DataStoreName=Toggle_Pin
  Equal : RelationalOperator  Operator=~=  OutDataTypeStr=boolean  RndMeth=Simplest
  Equal1 : RelationalOperator  Operator=~=  OutDataTypeStr=boolean  RndMeth=Simplest
  Equal2 : RelationalOperator  Operator=~=  OutDataTypeStr=boolean  RndMeth=Simplest
  NOT : Logic  Operator=NOT  IconShape=distinctive  AllPortsSameDT=off  OutDataTypeStr=boolean
  NOT1 : Logic  Operator=NOT  IconShape=distinctive  AllPortsSameDT=off  OutDataTypeStr=boolean
  NOT2 : Logic  Operator=NOT  IconShape=distinctive  AllPortsSameDT=off  OutDataTypeStr=boolean
  Plus : Sum
  Plus1 : Sum
  Plus2 : Sum
  Switch1 : Switch  Criteria=u2 > Threshold
  Switch2 : Switch  Criteria=u2 > Threshold
  Switch3 : Switch  Criteria=u2 > Threshold
  Timeout Counter 1 DEBUG : Subsystem
  Timeout Counter 2 DEBUG : Subsystem
  Timeout Counter 3 DEBUG : Subsystem
  wires:
  Constant6/1 -> Plus/2
  Plus/1 -> Switch2/1
  Plus2/1 -> Switch3/1
  Plus1/1 -> Switch1/1
  NOT/1 -> AND/2
  Data Store Read7/1 -> Switch3/3
  NOT2/1 -> AND2/2
  Data Store Read2/1 -> NOT1/1
  Equal2/1 -> AND2/1
  Equal1/1 -> AND1/1
  Data Store Read6/1 -> Plus1/1
  Data Store Read8/1 -> Plus2/1
  Data Store Read3/1 -> NOT2/1
  Switch3/1 -> Data Store Write3/1  "Timeout_Board3"
  Switch2/1 -> Data Store Write1/1  "Timeout_Board1"
  Constant1/1 -> Plus1/2
  Data Store Read5/1 -> Plus/1
  Data Store Read1/1 -> NOT/1
  Data Store Read9/1 -> Equal/2
  NOT1/1 -> AND1/2
  AND2/1 -> Timeout Counter 3 DEBUG/1(Timeout), Switch3/2
  Constant2/1 -> Plus2/2
  Data Store Read/1 -> Switch2/3
  Constant4/1 -> Equal2/1
  AND1/1 -> Timeout Counter 2 DEBUG/1(Timeout), Switch1/2
  Data Store Read4/1 -> Switch1/3
  Data Store Read10/1 -> Equal1/2
  Constant/1 -> Equal/1
  Switch1/1 -> Data Store Write2/1  "Timeout_Board2"
  Data Store Read11/1 -> Equal2/2
  Equal/1 -> AND/1
  Constant3/1 -> Equal1/1
  AND/1 -> Timeout Counter 1 DEBUG/1(Timeout), Switch2/2
  Constant5/1 -> Data Store Write4/1

== system HANcoder_E407_GTSync_v4/HANcoder STM32 Target - E407-STM32 algorithm/Global Ticks Increment/CAN Management/Matrix Cycle Manager/COMP Task - New Master/New Master ==
  note: Post voting process
  note: Logic Analyzer - DEBUG
      | Start of COMP task
  note: Logic Analyzer - DEBUG
  Enable : EnablePort  PropagateVarSize=During execution
  Constant10 : Constant  Value=Slave_Role
  Constant3 : Constant  OutDataTypeStr=boolean
  Constant9 : Constant  Value=Master_Role
  Data Store Read : DataStoreRead  DataStoreName=Master_ID
  Data Store Read27 : DataStoreRead  DataStoreName=Board_ID
  Data Store Write : DataStoreWrite  DataStoreName=Reset_Board
  Data Store Write1 : DataStoreWrite  DataStoreName=New_Master
  Data Store Write13 : DataStoreWrite  DataStoreName=Master_ID
  Data Store Write15 : DataStoreWrite  DataStoreName=Role_ID
  Data Store Write3 : DataStoreWrite  DataStoreName=Toggle_Pin
  Equal : RelationalOperator  Operator=~=  OutDataTypeStr=boolean  RndMeth=Simplest
  Equal6 : RelationalOperator  Operator===  OutDataTypeStr=boolean  RndMeth=Simplest
  Switch16 : Switch  Criteria=u2 > Threshold
  Votes recount to choose Master : Subsystem
  wires:
  Equal6/1 -> Switch16/2
  Data Store Read27/1 -> Equal6/2
  Switch16/1 -> Data Store Write15/1  "Role_ID_s"
  Constant9/1 -> Switch16/1
  Constant10/1 -> Switch16/3
  Data Store Read/1 -> Equal/1
  Equal/1 -> Data Store Write1/1
  Votes recount to choose Master/1(Master_ID_s) -> Equal6/1, Equal/2, Data Store Write13/1
  Votes recount to choose Master/2(Reset Board) -> Data Store Write/1
  Constant3/1 -> Data Store Write3/1

== system HANcoder_E407_GTSync_v4/HANcoder STM32 Target - E407-STM32 algorithm/Global Ticks Increment/CAN Management/Matrix Cycle Manager/COMP Task - Reset Board/RESET Board - Return to initialization ==
  note: Role reset
  note: CAN Rx preparation for sync
  note: Reset board state
  note: Logic Analyzer - DEBUG
      | Start of COMP task
  note: Logic Analyzer - DEBUG
  Enable : EnablePort
  Cast : DataTypeConversion  OutDataTypeStr=boolean
  Cast6 : DataTypeConversion  OutDataTypeStr=uint8
  Constant : Constant  Value=0
  Constant1 : Constant  Value=Sync_ID  OutDataTypeStr=uint32
  Constant3 : Constant  OutDataTypeStr=boolean
  Data Store Write : DataStoreWrite  DataStoreName=Reset_Board
  Data Store Write1 : DataStoreWrite  DataStoreName=New_Msg_Ready
  Data Store Write2 : DataStoreWrite  DataStoreName=Initialization_flag
  Data Store Write3 : DataStoreWrite  DataStoreName=RxID_buffer
  Data Store Write4 : DataStoreWrite  DataStoreName=Role_ID
  Data Store Write5 : DataStoreWrite  DataStoreName=Master_ID
  Data Store Write6 : DataStoreWrite  DataStoreName=Rx_State
  Data Store Write7 : DataStoreWrite  DataStoreName=Toggle_Pin
  NOT : Logic  Operator=NOT  IconShape=distinctive  AllPortsSameDT=off  OutDataTypeStr=boolean
  wires:
  Constant/1 -> Data Store Write5/1, Data Store Write4/1, Cast6/1, Cast/1
  Cast/1 -> Data Store Write1/1, NOT/1, Data Store Write/1
  NOT/1 -> Data Store Write2/1
  Constant1/1 -> Data Store Write3/1
  Cast6/1 -> Data Store Write6/1
  Constant3/1 -> Data Store Write7/1

== system HANcoder_E407_GTSync_v4/HANcoder STM32 Target - E407-STM32 algorithm/Global Ticks Increment/CAN Management/Matrix Cycle Manager/COMP Task - Reset Variables BC0/Reset variables ==
  note: Reset variables
  note: Logic Analyzer - DEBUG
      | Start of COMP task
  note: Logic Analyzer - DEBUG
  Enable : EnablePort
  Cast : DataTypeConversion  OutDataTypeStr=boolean
  Constant : Constant  Value=0
  Constant3 : Constant  OutDataTypeStr=boolean
  Data Store Write1 : DataStoreWrite  DataStoreName=sync_processed
  Data Store Write16 : DataStoreWrite  DataStoreName=votes  DataStoreElements=votes.First_Board#votes.Second_Board#votes.Third_Board
  Data Store Write2 : DataStoreWrite  DataStoreName=BC0_TM1_processed
  Data Store Write3 : DataStoreWrite  DataStoreName=BC0_TM2_processed
  Data Store Write4 : DataStoreWrite  DataStoreName=BC0_TM3_processed
  Data Store Write5 : DataStoreWrite  DataStoreName=Toggle_Pin
  wires:
  Constant/1 -> Data Store Write16/1, Cast/1, Data Store Write16/3, Data Store Write16/2
  Cast/1 -> Data Store Write4/1, Data Store Write3/1, Data Store Write2/1, Data Store Write1/1
  Constant3/1 -> Data Store Write5/1

== system HANcoder_E407_GTSync_v4/HANcoder STM32 Target - E407-STM32 algorithm/Global Ticks Increment/CAN Management/Matrix Cycle Manager/COMP Task - Reset Variables BC1/Reset Variables ==
  note: Reset variables
  note: Logic Analyzer - DEBUG
      | Start of COMP task
  note: Logic Analyzer - DEBUG
  Enable : EnablePort
  Cast : DataTypeConversion  OutDataTypeStr=boolean
  Constant : Constant  Value=0
  Constant3 : Constant  OutDataTypeStr=boolean
  Data Store Write1 : DataStoreWrite  DataStoreName=sync_processed
  Data Store Write3 : DataStoreWrite  DataStoreName=Toggle_Pin
  wires:
  Constant/1 -> Cast/1
  Cast/1 -> Data Store Write1/1
  Constant3/1 -> Data Store Write3/1

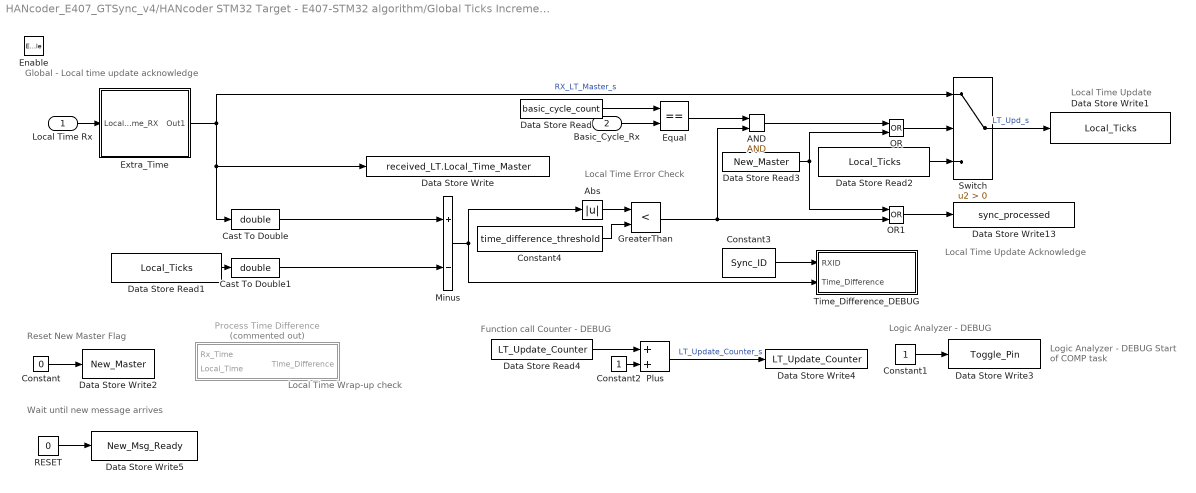
== system HANcoder_E407_GTSync_v4/HANcoder STM32 Target - E407-STM32 algorithm/Global Ticks Increment/CAN Management/Matrix Cycle Manager/COMP Task - Update LT/Local Time Update ==
  note: Function call Counter - DEBUG
  note: Reset New Master Flag
  note: Local Time Wrap-up check
  note: Local Time Error Check
  note: Local Time Update
  note: Local Time Update Acknowledge
  note: Global - Local time update acknowledge
  note: Logic Analyzer - DEBUG
      | Start of COMP task
  note: Logic Analyzer - DEBUG
  note: Wait until new message
      | arrives
  Local Time Rx : Inport
  Basic_Cycle_Rx : Inport  Port=2
  Enable : EnablePort
  AND : Logic  IconShape=distinctive  AllPortsSameDT=off  OutDataTypeStr=boolean
  Abs : Abs
  Cast To Double : DataTypeConversion  OutDataTypeStr=double
  Cast To Double1 : DataTypeConversion  OutDataTypeStr=double
  Constant : Constant  Value=0  OutDataTypeStr=boolean
  Constant1 : Constant  OutDataTypeStr=boolean
  Constant2 : Constant  OutDataTypeStr=int32
  Constant3 : Constant  Value=Sync_ID
  Constant4 : Constant  Value=time_difference_threshold
  Data Store Read : DataStoreRead  DataStoreName=basic_cycle_count
  Data Store Read1 : DataStoreRead  DataStoreName=Local_Ticks
  Data Store Read2 : DataStoreRead  DataStoreName=Local_Ticks
  Data Store Read3 : DataStoreRead  DataStoreName=New_Master
  Data Store Read4 : DataStoreRead  DataStoreName=LT_Update_Counter
  Data Store Write : DataStoreWrite  DataStoreName=received_LT  DataStoreElements=received_LT.Local_Time_Master
  Data Store Write1 : DataStoreWrite  DataStoreName=Local_Ticks  DataStoreElements=Local_Ticks
  Data Store Write13 : DataStoreWrite  DataStoreName=sync_processed
  Data Store Write2 : DataStoreWrite  DataStoreName=New_Master
  Data Store Write3 : DataStoreWrite  DataStoreName=Toggle_Pin
  Data Store Write4 : DataStoreWrite  DataStoreName=LT_Update_Counter
  Data Store Write5 : DataStoreWrite  DataStoreName=New_Msg_Ready
  Equal : RelationalOperator  Operator===  OutDataTypeStr=boolean  RndMeth=Simplest
  Extra_Time : Subsystem
  GreaterThan : RelationalOperator  Operator=<  OutDataTypeStr=boolean  RndMeth=Simplest
  Minus : Sum  Inputs=+-
  OR : Logic  Operator=OR  IconShape=distinctive  AllPortsSameDT=off  OutDataTypeStr=boolean
  OR1 : Logic  Operator=OR  IconShape=distinctive  AllPortsSameDT=off  OutDataTypeStr=boolean
  Plus : Sum
  Process Time Difference : Subsystem  Commented=on
  RESET : Constant  Value=0  OutDataTypeStr=boolean
  Switch : Switch  Criteria=u2 > Threshold
  Time_Difference_DEBUG : Subsystem
  wires:
  Constant3/1 -> Time_Difference_DEBUG/1(RXID)
  Minus/1 -> Time_Difference_DEBUG/2(Time_Difference), Abs/1
  Abs/1 -> GreaterThan/1
  Constant4/1 -> GreaterThan/2
  GreaterThan/1 -> AND/2, OR1/2
  Data Store Read1/1 -> Cast To Double1/1
  Data Store Read2/1 -> Switch/3
  Switch/1 -> Data Store Write1/1  "LT_Upd_s"
  AND/1 -> OR/1
  Data Store Read/1 -> Equal/1
  Equal/1 -> AND/1
  Basic_Cycle_Rx/1 -> Equal/2
  Cast To Double1/1 -> Minus/2
  Data Store Read3/1 -> OR/2, OR1/1
  OR/1 -> Switch/2
  OR1/1 -> Data Store Write13/1
  Constant/1 -> Data Store Write2/1
  Cast To Double/1 -> Minus/1
  Extra_Time/1(Out1) -> Switch/1, Data Store Write/1, Cast To Double/1  "RX_LT_Master_s"
  Local Time Rx/1 -> Extra_Time/1(Local_Time_RX)
  Constant1/1 -> Data Store Write3/1
  Data Store Read4/1 -> Plus/1
  Plus/1 -> Data Store Write4/1  "LT_Update_Counter_s"
  Constant2/1 -> Plus/2
  RESET/1 -> Data Store Write5/1

== system HANcoder_E407_GTSync_v4/HANcoder STM32 Target - E407-STM32 algorithm/Global Ticks Increment/CAN Management/Matrix Cycle Manager/COMP Task - Update LT1/Local Time Update ==
  note: Global - Local time update acknowledge
  note: Local Time Update Acknowledge
  note: Local Time Update
  note: Local Time Error Check
  note: Local Time Wrap-up check
  note: Reset New Master Flag
  note: Logic Analyzer - DEBUG
      | Start of COMP task
  note: Logic Analyzer - DEBUG
  Local Time Rx : Inport
  Basic_Cycle_Rx : Inport  Port=2
  Enable : EnablePort
  AND : Logic  IconShape=distinctive  AllPortsSameDT=off  OutDataTypeStr=boolean
  Abs : Abs
  Cast To Double : DataTypeConversion  OutDataTypeStr=double
  Cast To Double1 : DataTypeConversion  OutDataTypeStr=double
  Constant : Constant  Value=0  OutDataTypeStr=boolean
  Constant1 : Constant  OutDataTypeStr=boolean
  Constant3 : Constant  Value=Sync_ID
  Constant4 : Constant  Value=time_difference_threshold
  Data Store Read : DataStoreRead  DataStoreName=basic_cycle_count
  Data Store Read1 : DataStoreRead  DataStoreName=Local_Ticks
  Data Store Read2 : DataStoreRead  DataStoreName=Local_Ticks
  Data Store Read3 : DataStoreRead  DataStoreName=New_Master
  Data Store Write : DataStoreWrite  DataStoreName=received_LT  DataStoreElements=received_LT.Local_Time_Master
  Data Store Write1 : DataStoreWrite  DataStoreName=Local_Ticks
  Data Store Write13 : DataStoreWrite  DataStoreName=sync_processed
  Data Store Write2 : DataStoreWrite  DataStoreName=New_Master
  Data Store Write3 : DataStoreWrite  DataStoreName=Toggle_Pin
  Equal : RelationalOperator  Operator===  OutDataTypeStr=boolean  RndMeth=Simplest
  Extra_Time : Subsystem
  GreaterThan : RelationalOperator  Operator=<  OutDataTypeStr=boolean  RndMeth=Simplest
  Minus : Sum  Inputs=+-
  OR : Logic  Operator=OR  IconShape=distinctive  AllPortsSameDT=off  OutDataTypeStr=boolean
  OR1 : Logic  Operator=OR  IconShape=distinctive  AllPortsSameDT=off  OutDataTypeStr=boolean
  Process Time Difference : Subsystem  Commented=on
  RX-TX : Constant  Value=TM1-TM0  OutDataTypeStr=uint16
  Switch : Switch  Criteria=u2 > Threshold
  Time_Difference_DEBUG : Subsystem
  wires:
  Extra_Time/1(Out1) -> Switch/1, Cast To Double/1, Data Store Write/1
  Cast To Double/1 -> Minus/1
  Constant/1 -> Data Store Write2/1
  OR1/1 -> Data Store Write13/1
  OR/1 -> Switch/2
  Data Store Read3/1 -> OR1/1, OR/2
  Cast To Double1/1 -> Minus/2
  Basic_Cycle_Rx/1 -> Equal/2
  Equal/1 -> AND/1
  Data Store Read/1 -> Equal/1
  AND/1 -> OR/1
  Switch/1 -> Data Store Write1/1
  Data Store Read2/1 -> Switch/3
  Data Store Read1/1 -> Cast To Double1/1
  GreaterThan/1 -> OR1/2, AND/2
  Constant4/1 -> GreaterThan/2
  Abs/1 -> GreaterThan/1
  Minus/1 -> Abs/1, Time_Difference_DEBUG/2(Time_Difference)
  Constant3/1 -> Time_Difference_DEBUG/1(RXID)
  RX-TX/1 -> Extra_Time/2(RX_Update_Delay)
  Local Time Rx/1 -> Extra_Time/1(Local_Time_RX)
  Constant1/1 -> Data Store Write3/1
